simulink model "sim_model"  (Simulink 8.0)
settings: Solver=ode45  StartTime=0  StopTime=20  FixedStep=0.01  RelTol=1e-3
libraries: fmu_me_lib x1
settings Model: Creator=Tin Rabuzin  LastModifiedBy=Tin Rabuzin

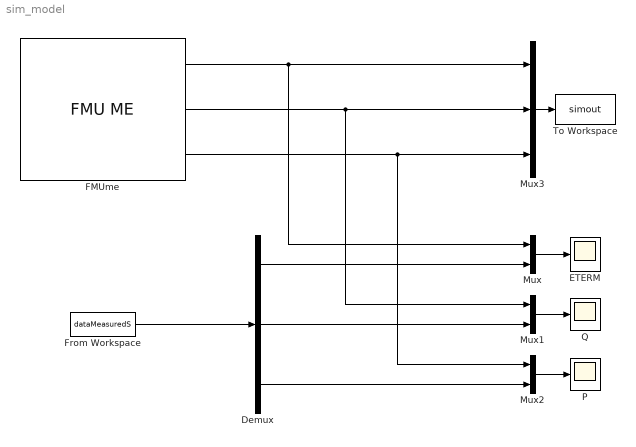
== system sim_model ==
  Demux : Demux  Outputs=3
  ETERM : Scope
      settings: TimeRange=20  YMin=1.05  YMax=1.06
  FMUme : fmu_me_lib/FMU ME  Description=Simulates an FMU for Model Exchange 1.0 or Model Exchange 2.0.
  From Workspace : FromWorkspace  VariableName=dataMeasuredS  SampleTime=0
  Mux : Mux  Inputs=2
  Mux1 : Mux  Inputs=2
  Mux2 : Mux  Inputs=2
  Mux3 : Mux  Inputs=3
  P : Scope
      settings: TimeRange=18  YMin=0.499  YMax=0.5015  SaveName=ScopeData2
  Q : Scope
      settings: YMin=0  YMax=2
  To Workspace : ToWorkspace  VariableName=simout  SampleTime=-1  SaveFormat=Structure With Time
  wires:
  From Workspace/1 -> Demux/1
  Demux/3 -> Mux2/2
  Demux/2 -> Mux1/2
  Demux/1 -> Mux/2
  Mux3/1 -> To Workspace/1
  Mux/1 -> ETERM/1
  Mux1/1 -> Q/1
  Mux2/1 -> P/1
  FMUme/1 -> Mux/1, Mux3/1
  FMUme/3 -> Mux2/1, Mux3/3
  FMUme/2 -> Mux1/1, Mux3/2
